simulink model "model_simulink"  (R2019a)
settings: Solver=VariableStepAuto  StartTime=0.0  StopTime=10.0  RelTol=1e-3
settings Model: Creator=KevinChng  LastModifiedBy=KevinChng
settings DebuggingCC: UnderSpecifiedDimensionMsg=warning

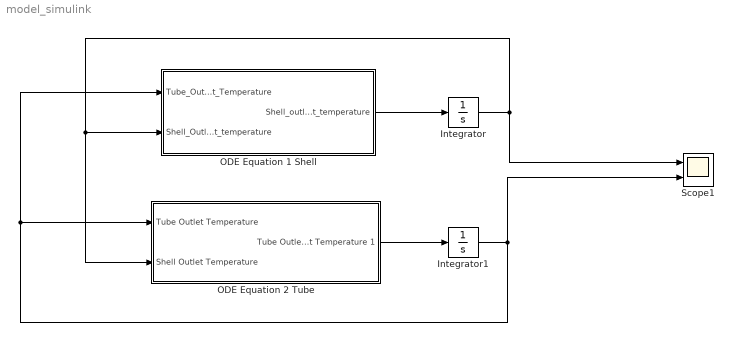
== system model_simulink ==
  Integrator : Integrator  InitialCondition=300
  Integrator1 : Integrator  InitialCondition=370
  ODE Equation 1 Shell : MATLAB Function  TreatAsAtomicUnit=on
  ODE Equation 2 Tube : Subsystem  TreatAsAtomicUnit=on
  Scope1 : Scope  NumInputPorts=2
  wires:
  ODE Equation 1 Shell/1(Shell_outlet_temperature) -> Integrator/1
  Integrator/1 -> ODE Equation 1 Shell/2(Shell_Outlet_temperature), ODE Equation 2 Tube/2(Shell Outlet Temperature), Scope1/1
  ODE Equation 2 Tube/1(Tube Outlet Temperature 1) -> Integrator1/1
  Integrator1/1 -> ODE Equation 2 Tube/1(Tube Outlet Temperature), ODE Equation 1 Shell/1(Tube_Outlet_Temperature), Scope1/2

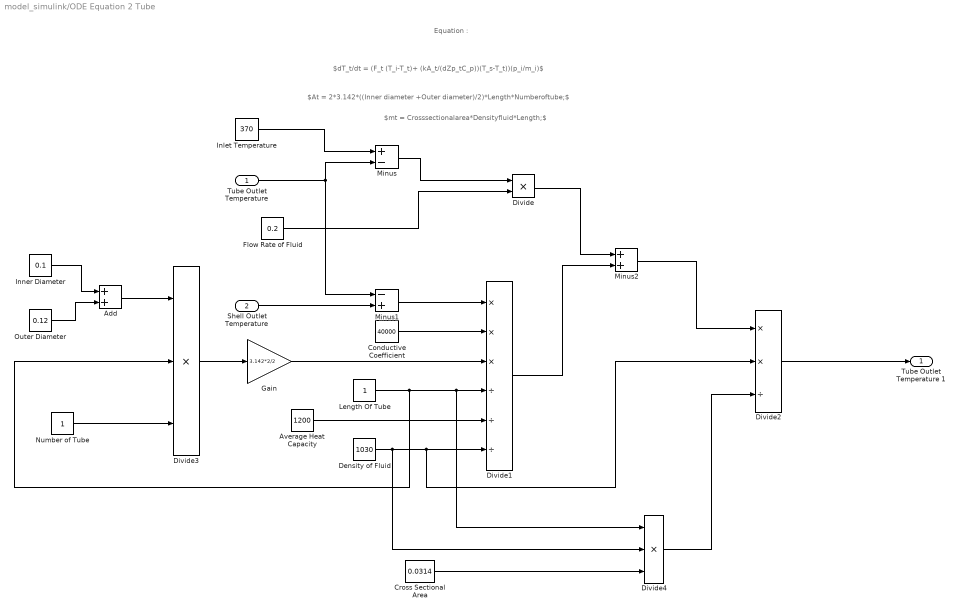
== system model_simulink/ODE Equation 2 Tube ==
  note: $mt = Crosssectionalarea*Densityfluid*Length;$
  note: Equation :
  note: $dT_t/dt = (F_t (T_i-T_t)+ (kA_t/(dZp_tC_p))(T_s-T_t))(p_i/m_i)$
  note: $At = 2*3.142*((Inner diameter +Outer diameter)/2)*Length*Numberoftube;$
  Tube Outlet Temperature : Inport
  Shell Outlet Temperature : Inport  Port=2
  Add : Sum
  Average Heat Capacity : Constant  Value=1200
  Conductive Coefficient : Constant  Value=40000
  Cross Sectional Area : Constant  Value=0.0314
  Density of Fluid : Constant  Value=1030  VectorParams1D=off  SampleTime=-1
  Divide : Product  Inputs=**
  Divide1 : Product  Inputs=***///
  Divide2 : Product  Inputs=**/
  Divide3 : Product  Inputs=***
  Divide4 : Product  Inputs=***
  Flow Rate of Fluid : Constant  Value=0.2
  Gain : Gain  Gain=3.142*2/2
  "Inlet Temperature " : Constant  Value=370
  Inner Diameter : Constant  Value=0.1
  Length Of Tube : Constant
  Minus : Sum  Inputs=+-
  Minus1 : Sum  Inputs=-+
  Minus2 : Sum
  Number of Tube : Constant
  Outer Diameter : Constant  Value=0.12
  Tube Outlet Temperature 1 : Outport
  wires:
  "Inlet Temperature "/1 -> Minus/1
  Tube Outlet Temperature/1 -> Minus/2, Minus1/1
  Minus/1 -> Divide/1
  Flow Rate of Fluid/1 -> Divide/2
  Shell Outlet Temperature/1 -> Minus1/2
  Minus1/1 -> Divide1/1
  Conductive Coefficient/1 -> Divide1/2
  Length Of Tube/1 -> Divide4/1, Divide1/4, Divide3/2
  Density of Fluid/1 -> Divide4/2, Divide2/2, Divide1/6
  Average Heat Capacity/1 -> Divide1/5
  Divide/1 -> Minus2/1
  Divide1/1 -> Minus2/2
  Minus2/1 -> Divide2/1
  Divide4/1 -> Divide2/3
  Divide2/1 -> Tube Outlet Temperature 1/1
  Gain/1 -> Divide1/3
  Divide3/1 -> Gain/1
  Inner Diameter/1 -> Add/1
  Outer Diameter/1 -> Add/2
  Add/1 -> Divide3/1
  Number of Tube/1 -> Divide3/3
  Cross Sectional Area/1 -> Divide4/3

== matlab function model_simulink/ODE Equation 1 Shell ==
  data: Tube_Outlet_Temperature input; Shell_outlet_temperature output; Shell_Outlet_temperature input
function Shell_outlet_temperature = fcn(Tube_Outlet_Temperature,Shell_Outlet_temperature)

% Constant
T_ambient = 30+273.15;
Inner_diameter_tube = 0.1;
Outer_diameter_tube = 0.12;
Length_tube = 1;
Number_tube = 1;
Inner_diameter_shell = 0.2;
Outer_diameter_shell = 0.22;
Conductive_heattransfer_tube_shell = 40000;
convective_heattransfer_shell_ambient = 500;
Cross_sectional_area_shell = 0.0254;
At = 2*3.142*((Inner_diameter_tube+Outer_diameter_tube)/2)*Length_tube*Number_tube;
Ad = 2*3.142*((Inner_diameter_shell+Outer_diameter_shell)/2)*Length_tube;
Average_heat_capacity_shell=4185;
Temperature_inlet_shell=26.8+273.15;
Density_fluid_shell = 1000;
Flow_rate_shell = 0.1;
ms = Cross_sectional_area_shell*Density_fluid_shell*Length_tube;


% Constant
Shell_outlet_temperature = ((Temperature_inlet_shell-Shell_Outlet_temperature)...
    - (Conductive_heattransfer_tube_shell*At)*(Shell_Outlet_temperature-Tube_Outlet_Temperature)/(Length_tube*Density_fluid_shell*Flow_rate_shell*Average_heat_capacity_shell)...
    - (convective_heattransfer_shell_ambient*Ad)*(Temperature_inlet_shell-T_ambient)/(Density_fluid_shell*Flow_rate_shell*Average_heat_capacity_shell))...
    * (Density_fluid_shell*Flow_rate_shell/ms);
